simulink model "zad1_a"  (R2020a)
settings: Solver=FixedStepDiscrete  StartTime=0.0  StopTime=0.0  RelTol=1e-3
libraries: CPOiS_SourcesSinks x6, CPOiS_HistogramOperations x1
settings Model: Creator=johnb  LastModifiedBy=johnb

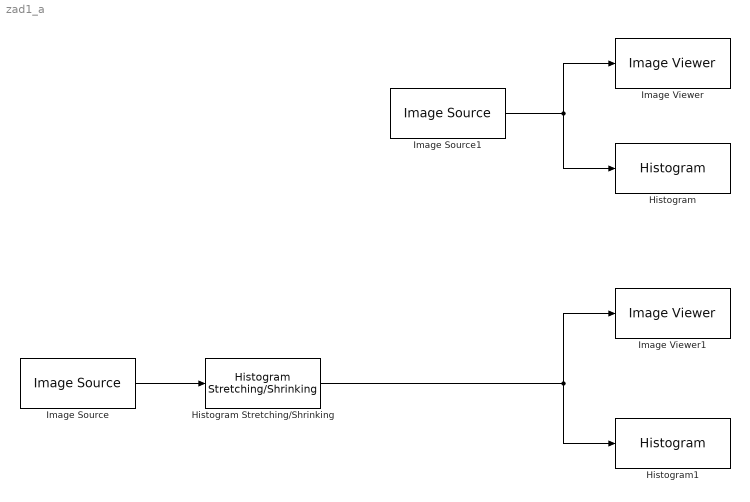
== system zad1_a ==
  Histogram : CPOiS_SourcesSinks/Histogram
      settings: SourceProductName=CPOiS - Digital image and signal processing
  Histogram Stretching/Shrinking : CPOiS_HistogramOperations/Histogram Stretching//Shrinking  minimum=64  maximum=191
      settings: SourceProductName=CPOiS - Digital image and signal processing
  Histogram1 : CPOiS_SourcesSinks/Histogram
      settings: SourceProductName=CPOiS - Digital image and signal processing
  Image Source : CPOiS_SourcesSinks/Image Source  FileSelection=airport.png
      settings: SourceProductName=CPOiS - Digital image and signal processing
  Image Source1 : CPOiS_SourcesSinks/Image Source  FileSelection=airport.png
      settings: SourceProductName=CPOiS - Digital image and signal processing
  Image Viewer : CPOiS_SourcesSinks/Image Viewer
      settings: SourceProductName=CPOiS - Digital image and signal processing
  Image Viewer1 : CPOiS_SourcesSinks/Image Viewer
      settings: SourceProductName=CPOiS - Digital image and signal processing
  wires:
  Image Source/1 -> Histogram Stretching/Shrinking/1
  Image Source1/1 -> Image Viewer/1, Histogram/1
  Histogram Stretching/Shrinking/1 -> Histogram1/1, Image Viewer1/1
